simulink subsystem "quarter_suspension"  (R2024b)
settings: Solver=VariableStepAuto  StartTime=0.0  StopTime=10.0  RelTol=1e-3
model mask{radius=1, spin_inertia=1, offset=[0; 0; 0], ride_rate=1, damp_rate=0, C_i=0, C_a=0, min_velocity=0, initial_spin=0}
  mask prompts: radius "Wheel radius [m]"; spin_inertia "Wheel inertia [kg m²]"; offset "Resting point offset [m]"; ride_rate "Ride rate [N/m]"; damp_rate "Daming rate [N/(m/s)]"; C_i "Traction coefficient [N]"; C_a "Sideslip coefficient [N]"; min_velocity "Minimum velocity [m/s]"; initial_spin "Initial spin [rad/s]"
libraries: aerolibutil x7, matrix_library x2
settings Model: Creator=yevge  LastModifiedBy=Yevgeniy Gorbachev

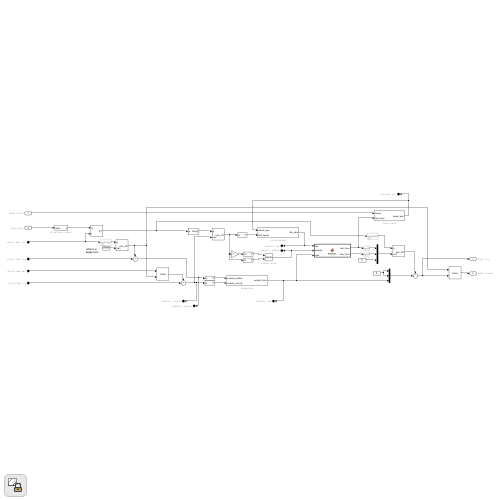
[thumbnail: Simulink's stored preview of the top-level diagram]
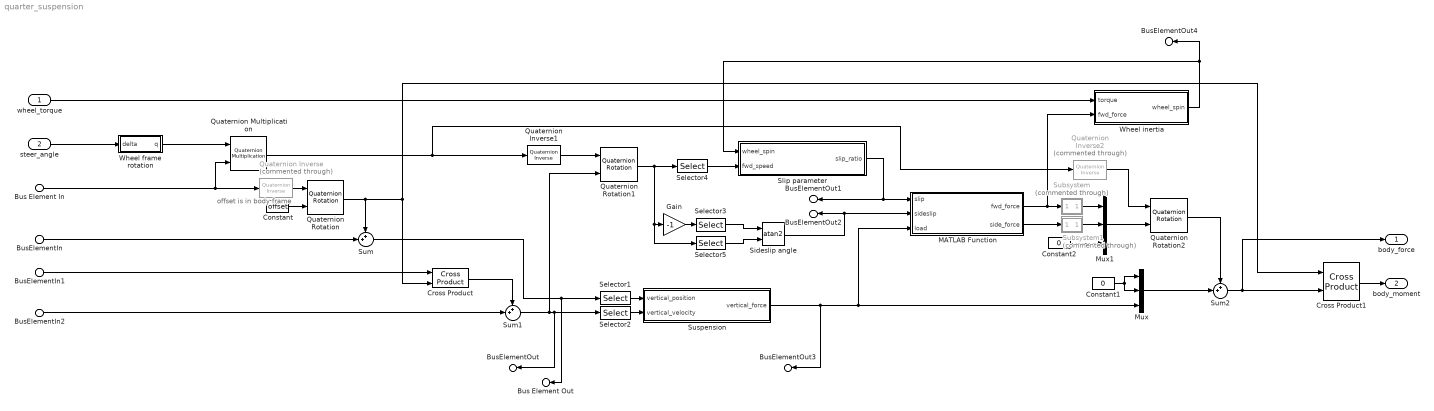
== system quarter_suspension ==
  note: offset is in body frame
  wheel_torque : Inport  Unit=N*m@torque
  steer_angle : Inport  Port=2
  Bus Element In : Inport  Port=3  PortName=vehicle_data  Element=ornt
  BusElementIn : Inport  Port=3  PortName=vehicle_data  Element=pos
  BusElementIn1 : Inport  Port=3  PortName=vehicle_data  Element=spin
  BusElementIn2 : Inport  Port=3  PortName=vehicle_data  Element=vel
  Constant : Constant  Value=offset
  Constant1 : Constant  Value=0
  Constant2 : Constant  Value=0
  Cross Product : matrix_library/Cross Product
  Cross Product1 : matrix_library/Cross Product
  Gain : Gain  Gain=-1
  MATLAB Function : MATLAB Function  TreatAsAtomicUnit=on
  Mux : Mux  Inputs=3
  Mux1 : Mux  Inputs=3
  Quaternion Inverse : aerolibutil/Quaternion Inverse  Commented=through
  Quaternion Inverse1 : aerolibutil/Quaternion Inverse
  Quaternion Inverse2 : aerolibutil/Quaternion Inverse  Commented=through
  Quaternion Multiplication : aerolibutil/Quaternion Multiplication
  Quaternion Rotation : aerolibutil/Quaternion Rotation
  Quaternion Rotation1 : aerolibutil/Quaternion Rotation
  Quaternion Rotation2 : aerolibutil/Quaternion Rotation
  Selector1 : Selector  InputPortWidth=3  IndexOptions=Index vector (dialog)  Indices=3  OutputSizes=1
  Selector2 : Selector  InputPortWidth=3  IndexOptions=Index vector (dialog)  Indices=3  OutputSizes=1
  Selector3 : Selector  InputPortWidth=3  IndexOptions=Index vector (dialog)  Indices=2  OutputSizes=1
  Selector4 : Selector  InputPortWidth=3  IndexOptions=Index vector (dialog)  Indices=1  OutputSizes=1
  Selector5 : Selector  InputPortWidth=3  IndexOptions=Index vector (dialog)  Indices=1  OutputSizes=1
  Sideslip angle : Trigonometry  Operator=atan2
  Slip parameter : Subsystem
  Subsystem : Subsystem  Commented=through
  Subsystem1 : Subsystem  Commented=through
  Sum : Sum  Inputs=++|
  Sum1 : Sum  Inputs=++|
  Sum2 : Sum  Inputs=++|
  Suspension : Subsystem
  Wheel frame rotation : Subsystem
  Wheel inertia : Subsystem
  body_force : Outport  Unit=N  PortDimensions=[3 1]
  body_moment : Outport  Port=2  Unit=N*m  PortDimensions=[3 1]
  Bus Element Out : Outport  Port=3  PortName=telemetry  Element=position
  BusElementOut : Outport  Port=3  PortName=telemetry  Element=velocity
  BusElementOut1 : Outport  Port=3  PortName=telemetry  Element=slip
  BusElementOut2 : Outport  Port=3  PortName=telemetry  Element=sideslip
  BusElementOut3 : Outport  Port=3  PortName=telemetry  Element=load
  BusElementOut4 : Outport  Port=3  PortName=telemetry  Element=spin
  wires:
  steer_angle/1 -> Wheel frame rotation/1(delta)
  Bus Element In/1 -> Quaternion Inverse/1, Quaternion Multiplication/2
  Quaternion Inverse/1 -> Quaternion Rotation/1
  Constant/1 -> Quaternion Rotation/2
  Quaternion Rotation/1 -> Sum/1, Cross Product1/1, Cross Product/2
  Cross Product/1 -> Sum1/1
  wheel_torque/1 -> Wheel inertia/1(torque)
  Sum/1 -> Bus Element Out/1, Selector1/1
  Sum1/1 -> Quaternion Rotation1/2, BusElementOut/1, Selector2/1
  Constant1/1 -> Mux/2, Mux/1
  Cross Product1/1 -> body_moment/1
  BusElementIn/1 -> Sum/2
  BusElementIn1/1 -> Cross Product/1
  BusElementIn2/1 -> Sum1/2
  Wheel inertia/1(wheel_spin) -> Slip parameter/1(wheel_spin), BusElementOut4/1
  Quaternion Inverse1/1 -> Quaternion Rotation1/1
  Selector4/1 -> Slip parameter/2(fwd_speed)
  Selector1/1 -> Suspension/1(vertical_position)
  Selector2/1 -> Suspension/2(vertical_velocity)
  Selector3/1 -> Sideslip angle/1
  Selector5/1 -> Sideslip angle/2
  Quaternion Rotation1/1 -> Selector5/1, Gain/1, Selector4/1
  Slip parameter/1(slip_ratio) -> MATLAB Function/1(slip), BusElementOut1/1
  MATLAB Function/1(fwd_force) -> Subsystem/1(fwd_force), Wheel inertia/2(fwd_force)
  Quaternion Multiplication/1 -> Quaternion Inverse2/1, Quaternion Inverse1/1
  Sum2/1 -> body_force/1, Cross Product1/2
  Mux/1 -> Sum2/2
  Mux1/1 -> Quaternion Rotation2/2
  Quaternion Inverse2/1 -> Quaternion Rotation2/1
  Quaternion Rotation2/1 -> Sum2/1
  Suspension/1(vertical_force) -> BusElementOut3/1, MATLAB Function/3(load), Mux/3
  Constant2/1 -> Mux1/3
  MATLAB Function/2(side_force) -> Subsystem1/1(fwd_force)
  Subsystem/1(Out1) -> Mux1/1
  Subsystem1/1(Out1) -> Mux1/2
  Sideslip angle/1 -> MATLAB Function/2(sideslip), BusElementOut2/1
  Wheel frame rotation/1(q) -> Quaternion Multiplication/1
  Gain/1 -> Selector3/1

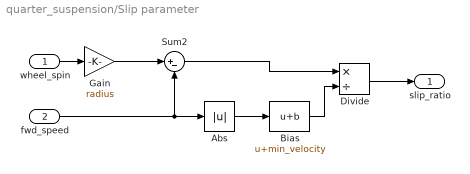
== system quarter_suspension/Slip parameter ==
  wheel_spin : Inport
  fwd_speed : Inport  Port=2
  Abs : Abs  SaturateOnIntegerOverflow=off
  Bias : Bias  Bias=min_velocity  SaturateOnIntegerOverflow=off
  Divide : Product  Inputs=*/
  Gain : Gain  Gain=radius
  Sum2 : Sum  Inputs=|+-
  slip_ratio : Outport
  wires:
  Abs/1 -> Bias/1
  Sum2/1 -> Divide/1
  Bias/1 -> Divide/2
  fwd_speed/1 -> Sum2/2, Abs/1
  Gain/1 -> Sum2/1
  Divide/1 -> slip_ratio/1
  wheel_spin/1 -> Gain/1

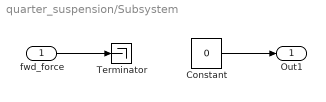
== system quarter_suspension/Subsystem ==
  fwd_force : Inport
  Constant : Constant  Value=0
  Terminator : Terminator
  Out1 : Outport
  wires:
  Constant/1 -> Out1/1
  fwd_force/1 -> Terminator/1

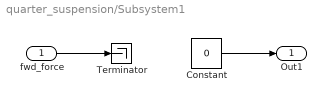
== system quarter_suspension/Subsystem1 ==
  fwd_force : Inport
  Constant : Constant  Value=0
  Terminator : Terminator
  Out1 : Outport
  wires:
  Constant/1 -> Out1/1
  fwd_force/1 -> Terminator/1

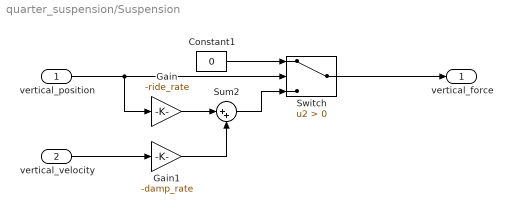
== system quarter_suspension/Suspension ==
  vertical_position : Inport
  vertical_velocity : Inport  Port=2
  Constant1 : Constant  Value=0
  Gain : Gain  Gain=-ride_rate
  Gain1 : Gain  Gain=-damp_rate
  Sum2 : Sum  Inputs=|++
  Switch : Switch  Criteria=u2 > Threshold  SaturateOnIntegerOverflow=off  InputSameDT=off
  vertical_force : Outport
  wires:
  vertical_position/1 -> Gain/1, Switch/2
  Gain/1 -> Sum2/1
  vertical_velocity/1 -> Gain1/1
  Gain1/1 -> Sum2/2
  Sum2/1 -> Switch/3
  Constant1/1 -> Switch/1
  Switch/1 -> vertical_force/1

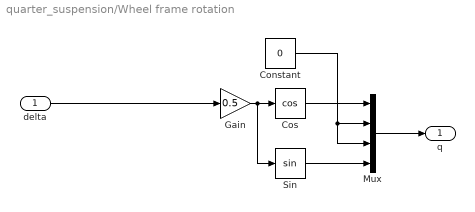
== system quarter_suspension/Wheel frame rotation ==
  delta : Inport
  Constant : Constant  Value=0
  Cos : Trigonometry  Operator=cos
  Gain : Gain  Gain=0.5
  Mux : Mux
  Sin : Trigonometry
  q : Outport
  wires:
  Sin/1 -> Mux/4
  delta/1 -> Gain/1
  Constant/1 -> Mux/3, Mux/2
  Mux/1 -> q/1
  Cos/1 -> Mux/1
  Gain/1 -> Sin/1, Cos/1

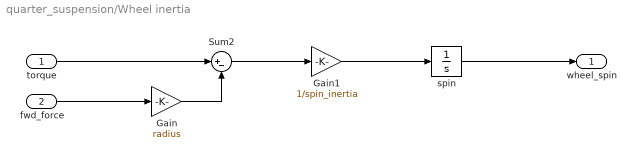
== system quarter_suspension/Wheel inertia ==
  torque : Inport
  fwd_force : Inport  Port=2
  Gain : Gain  Gain=radius
  Gain1 : Gain  Gain=1/spin_inertia
  Sum2 : Sum  Inputs=|+-
  spin : Integrator  InitialCondition=initial_spin  ContinuousStateAttributes='spin'
  wheel_spin : Outport
  wires:
  Sum2/1 -> Gain1/1
  torque/1 -> Sum2/1
  Gain/1 -> Sum2/2
  Gain1/1 -> spin/1
  fwd_force/1 -> Gain/1
  spin/1 -> wheel_spin/1

== matlab function quarter_suspension/MATLAB Function ==
  data: slip input; fwd_force output; sideslip input; load input; side_force output
function [fwd_force, side_force] = traction(slip, sideslip, load) 
    fwd_force = sin(atan(slip)) * load;
    side_force = sin(tan(sideslip)) * load;
end
